simulink model "verify_HouseSimple_mdl"  (R2018b)
settings: Solver=ode45  StartTime=0  StopTime=365*24*3600  RelTol=1e-3  EnableMultiTasking=on
InitFcn:
  | load('DE_TRY2010_04_averageYear')
undefined symbols (not defined in the file or in its folder): path_carnot
libraries: carnot x4
settings Model: SimulationMode=accelerator  Creator=drhf  LastModifiedBy=drhf
settings DataIOCC: SaveFormat=Array  SignalLoggingSaveFormat=ModelDataLogs
settings OptimizationCC: ExpressionDepthLimit=2147483647  LifeSpan=inf
settings DebuggingCC: UnderspecifiedInitializationDetection=Classic  MergeDetectMultiDrivingBlocksExec=none  SolverPrmCheckMsg=warning  FcnCallInpInsideContextMsg=warning  StateNameClashWarn=warning  SFUnexpectedBacktrackingDiag=warning  SFNoUnconditionalDefaultTransitionDiag=warning  SFExecutionAtInitializationDiag=none
settings HardwareCC: ProdBitPerPointer=32  ProdBitPerSizeT=32  ProdBitPerPtrDiffT=32  ProdLargestAtomicFloat=None  ProdIntDivRoundTo=Undefined  ProdEndianess=Unspecified  ProdWordSize=32  ProdHWDeviceType=32-bit Generic
settings ModelReferenceCC: PropagateSignalLabelsOutOfModel=off
settings SFSimCC: SimUseLocalCustomCode=off
settings RTWCC: RTWUseLocalCustomCode=off
settings CodeAppCC: StateflowObjectComments=on
settings GRTTargetCC: TargetLangStandard=C89/C90 (ANSI)  GeneratePreprocessorConditionals=Disable all  CombineOutputUpdateFcns=off  GRTInterface=on
settings ConfigComp: CovMetricSettings=dw  CovHtmlReporting=on  CovSaveCumulativeToWorkspaceVar=on  CovSaveSingleToWorkspaceVar=on  CovExternalEMLEnable=off

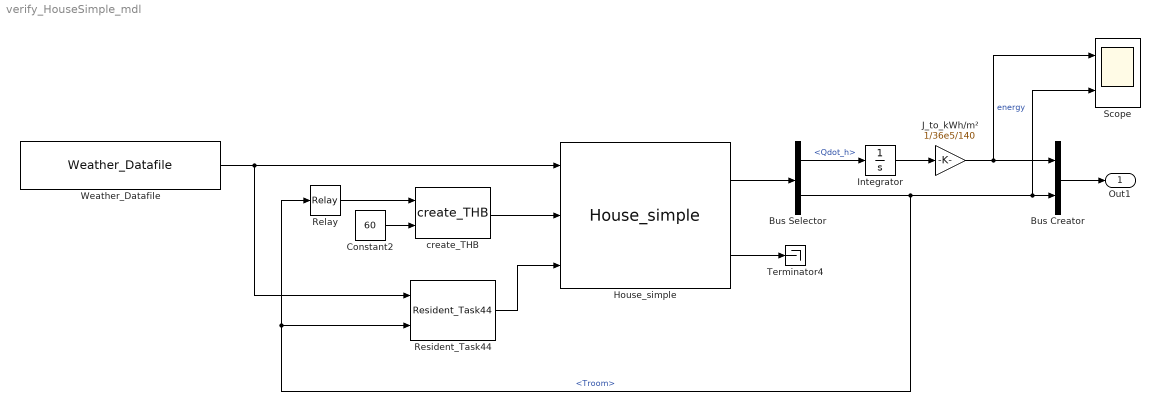
== system verify_HouseSimple_mdl ==
  Bus Creator : BusCreator  Inputs=2
  Bus Selector : BusSelector  OutputSignals=Qdot.Qdot_h,Troom
  Constant2 : Constant  Value=60
  House_simple : carnot/Load/Houses/House_simple  tini=20  dtroom=inf  Tmeaninside=23.8  deltathetai=3.8  Tmeanoutside=11  deltathetae=9.3  tshift=319*3600  PathName=fullfile(path_carnot('libsl'), 'Load', 'Houses', 'House_simple', 'parameter_set')  FileName='Default_HouseSimple.mat'  userPath=off  userParam=off  Ahabit=140  Hroom=2.5  slabwidth=10  slablength=7  dwall=0.4  UAwall=100  capa=500000  utot=0.183  gammat=0  cond_ground=2  cp_ground=800  rho_ground=2500  Awindow=[12 4 3 4]  AziWin=[0 90 -180 -90]  Uwindow=[2 2 2 2]  Gwindow=[0.5 0.5 0.5 0.5]  alpha=10  H=1.2  W=1  Nwin=4  Ventilationrate=0.4  Heatrecovery=0  pnom=10000  dtnom=49.83  expo=1.3  mcap=10*4812  lin=100  qua=100
      settings: SourceProductName=Carnot
  Integrator : Integrator
  J_to_kWh/m² : Gain  Gain=1/36e5/140
  Relay : Relay  OnSwitchValue=20.1  OffSwitchValue=19.9  OnOutputValue=0  OffOutputValue=800/3600
  Resident_Task44 : carnot/Load/Houses/Resident_Task44  period=24*3600  rep_seq_te=[0 1 6 7 8 9 11 12 13 18 19 20 22 23]*3600  rep_seq_de=[1 5 1 1 1 2 1 1 4 2 1 2 1 1]*3600  rep_seq_ye=[105 55 392.5 457.5 420 55 250 55 120 170 615 420 442.5 355]  rep_seq_to=[0 6 7 8 9 11 12 13 14 15 17 18 20 21 22]*3600  rep_seq_do=[6 1 1 1 2 1 1 1 1 2 1 2 1 1 2]*3600  rep_seq_yo=[4 2 3 2 0 1 3 2 1 0 1 2 4 3 4]*60  Topen=24  Tclose=23  TrAboveTa=2  TaTooCold=12  timeFIR=24  TaIni=12  starttime=8  stoptime=22  TroomShadeOn=23.8  TroomShadeOff=22.8  SolarShadeOn=300  SolarShadeOff=200  max_shade=1  CalcAirComp=off  mdotCO2=0  mdotH2O=0  mdotVOC=0
      settings: SourceProductName=Carnot
  Scope : Scope  NumInputPorts=2
  Terminator4 : Terminator
  Weather_Datafile : carnot/Weather/Weather_Datafile  PathName=path_carnot('data')  FileName='DE_TRY2010_04_averageYear.mat'  UserParam=off  VariableName=DE_TRY2010_04_averageYear  SampleTime=3600
      settings: SourceProductName=Carnot
  create_THB : carnot/Source/Simple/create_THB  p=1e5  fluid=Water  mix=0  mix2=0  mix3=0  dia=0.02  hgt=0  mID=No Pressure Drop
      settings: SourceProductName=Carnot
  Out1 : Outport
  wires:
  Weather_Datafile/1 -> Resident_Task44/1, House_simple/1
  Bus Creator/1 -> Out1/1
  House_simple/2 -> Terminator4/1
  House_simple/1 -> Bus Selector/1
  Bus Selector/2 -> Resident_Task44/2, Relay/1, Bus Creator/2, Scope/2  "<Troom>"
  Constant2/1 -> create_THB/2
  Relay/1 -> create_THB/1
  create_THB/1 -> House_simple/2
  Bus Selector/1 -> Integrator/1  "<Qdot_h>"
  Integrator/1 -> J_to_kWh/m²/1
  J_to_kWh/m²/1 -> Scope/1, Bus Creator/1  "energy"
  Resident_Task44/1 -> House_simple/3
